simulink model "WWmodel1"  (R2021b)
settings: Solver=VariableStepAuto  StartTime=0.0  StopTime=10.0  RelTol=1e-3
settings Model: Creator=Studenci  LastModifiedBy=Studenci

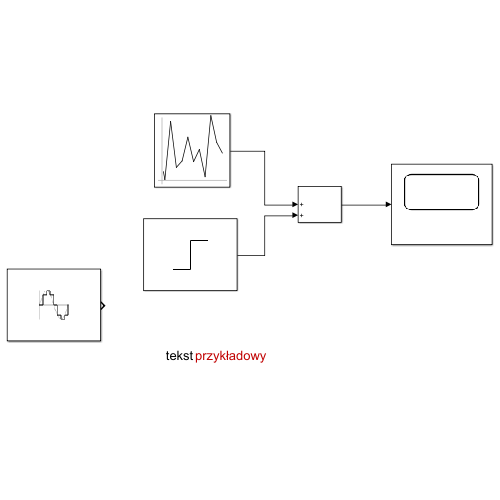
[thumbnail: Simulink's stored preview of the top-level diagram]
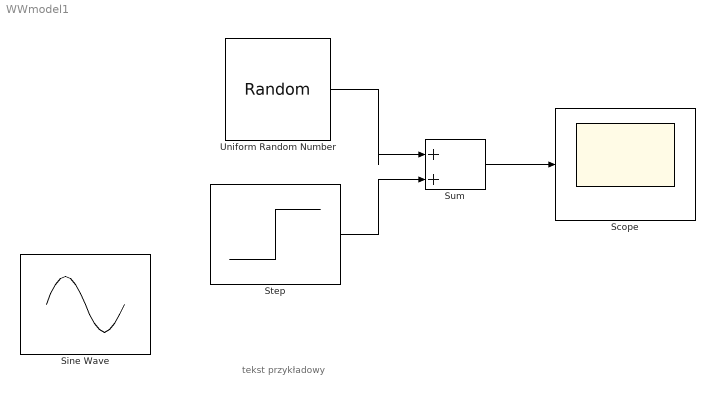
== system WWmodel1 ==
  note: tekst przykładowy
  Scope : Scope
  Sine Wave : Sin  Amplitude=10  Bias=10  Frequency=100000  Phase=2  SampleTime=100000000
  Step : Step  Time=2  After=5  SampleTime=0
  Sum : Sum  Inputs=|++
  Uniform Random Number : UniformRandomNumber  Minimum=0  Maximum=5  SampleTime=1
  wires:
  Step/1 -> Sum/2
  Sum/1 -> Scope/1
  Uniform Random Number/1 -> Sum/1
